simulink model "traffic_Light"  (R2018a)
settings: Solver=FixedStepDiscrete  StartTime=0.0  StopTime=inf  RelTol=1e-3
settings Model: Creator=Ayman_Elgammal  LastModifiedBy=Ayman_Elgammal
settings OptimizationCC: DefaultParameterBehavior=Inlined  EnhancedBackFolding=on  PassReuseOutputArgsAs=Individual arguments  OptimizeBlockOrder=speed  DifferentSizesBufferReuse=on  OptimizationCustomize=off
settings DebuggingCC: UnderspecifiedInitializationDetection=Classic  MergeDetectMultiDrivingBlocksExec=none  ParameterTunabilityLossMsg=error  LibraryContextMissingDiagnostic=warning
settings ModelReferenceCC: PropagateSignalLabelsOutOfModel=off
settings SFSimCC: SimUseLocalCustomCode=on  MATLABDynamicMemAlloc=off
settings RTWCC: SystemTargetFile=ert.tlc  GenCodeOnly=on  TemplateMakefile=ert_default_tmf  GenerateReport=on  RTWUseLocalCustomCode=on  IncludeHyperlinkInReport=on  LaunchReport=on  GenerateTraceInfo=on  GenerateTraceReport=on  GenerateTraceReportSl=on  GenerateTraceReportSf=on  GenerateTraceReportEml=on
settings CodeAppCC: ForceParamTrailComments=on  IgnoreCustomStorageClasses=off  OperatorAnnotations=on  SimulinkDataObjDesc=on  SFDataObjDesc=on  InsertBlockDesc=on
settings ERTTargetCC: TargetLangStandard=C99 (ISO)  GenerateSampleERTMain=on  InlinedParameterPlacement=NonHierarchical  ERTCustomFileTemplate=example_file_process.tlc

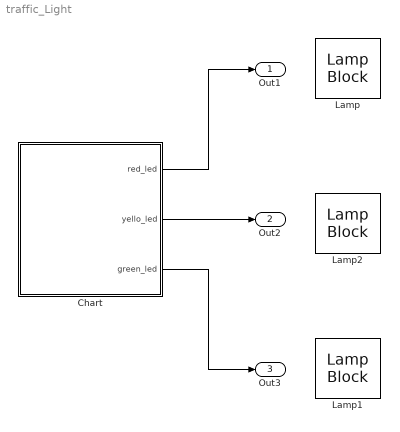
== system traffic_Light ==
  Chart : Stateflow chart  TreatAsAtomicUnit=on
  Lamp : LampBlock  WebBlockId=2
  Lamp1 : LampBlock  WebBlockId=3
  Lamp2 : LampBlock  WebBlockId=4
  Out1 : Outport
  Out2 : Outport  Port=2
  Out3 : Outport  Port=3
  wires:
  Chart/1(red_led) -> Out1/1
  Chart/2(yello_led) -> Out2/1
  Chart/3(green_led) -> Out3/1

== stateflow chart traffic_Light/Chart ==
  state go
    en:
    du:
    yello_led=0;
    red_led=0;
    green_led=1;
    ex:
  state ready
    en:
    red_led=0;
    green_led=0;
    yello_led=0;
    du:
    yello_led=1;
    red_led=0;
    green_led=0;
    ex:
  state stop
    en:
    du:
    yello_led=0;
    red_led=1;
    green_led=0;
    ex:
  (default) -> ready
  go -> ready : after(3000,msec)
  ready -> stop : after(3000,msec)
  stop -> go : after(3000,msec)
  data: green_led local uint8; yello_led local uint8; red_led local uint8; green_led local uint8; yello_led local uint8; red_led local uint8; green_led local uint8; yello_led local uint8; red_led local uint8; red_led output uint8; yello_led output uint8; green_led output uint8
